simulink model "freqScope"  (R2015a)
settings: Solver=ode45  StartTime=0.0  StopTime=1  RelTol=1e-3
values from neighbouring files (symbols this model uses):
  Fs = 48000    [ex1_1.m]    (also in ex1_2.m; lab1_1.m; lab1_2.m)
undefined symbols (not defined in the file or in its folder): get
libraries: dspspect3 x1, dspsnks4 x1
settings Model: CovSFcnEnable=off  Creator=davidding  LastModifiedBy=kwongr
settings DebuggingCC: SolverPrmCheckMsg=warning

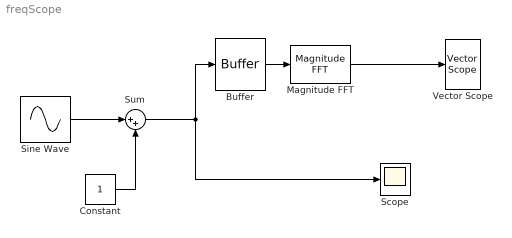
== system freqScope ==
  Buffer : Buffer  N=256  TreatMby1Signals=One channel
  Constant : Constant  SampleTime=1/48000
  Magnitude FFT : dspspect3/Magnitude FFT  mag_or_magsq=Magnitude squared  FFTImplementation=Auto  fftLenInherit=off  fftsize=256  WrapInput=on
  Scope : Scope
      settings: TimeRange=0.02744003816738705
  Sine Wave : Sin  SineType=Sample based  Samples=48  SampleTime=1/48000
  Sum : Sum  Inputs=|++
  Vector Scope : dspsnks4/Vector Scope  ScopeProperties=on  Domain=Frequency  HorizSpan=1  DisplayProperties=off  AxisGrid=on  Memory=off  FrameNumber=on  AxisLegend=off  AxisZoom=off  OpenScopeAtSimStart=on  OpenScopeImmediately=off  FigPos=get(0,'defaultfigureposition')  AxisProperties=off  XUnits=Hertz  XRange=[-Fs/2...Fs/2]  InheritXIncr=on  XIncr=1  XLabel=Time  XLimit=Auto  XMin=0  XMax=1  XStart=0  YUnits=dB  YLabel=Amplitude  LineProperties=off  XAxisParamsVer=6.9
      settings: YMin=-10  YMax=100
  wires:
  Sine Wave/1 -> Sum/1
  Constant/1 -> Sum/2
  Sum/1 -> Scope/1, Buffer/1
  Magnitude FFT/1 -> Vector Scope/1
  Buffer/1 -> Magnitude FFT/1
